simulink model "l1"  (R2016a)
settings: Solver=ode23  StartTime=0.0  StopTime=1000  RelTol=1e-10
settings Model: Creator=wojta  LastModifiedBy=wojta

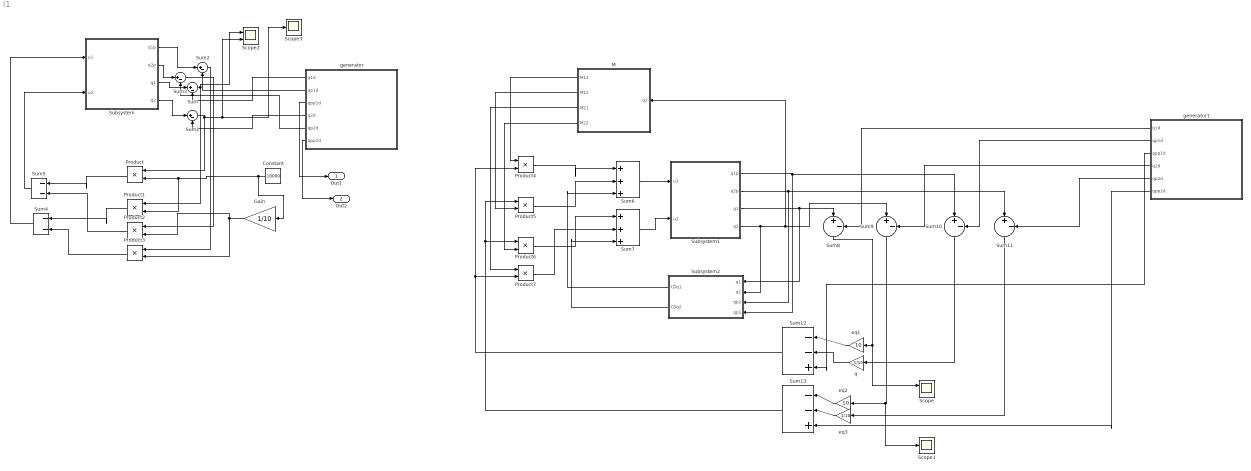
== system l1 ==
  Constant : Constant  Value=10000
  Gain : Gain  Gain=1/10
  M : Subsystem
  Product{,1..7} (8 alike) : Product
  Scope : Scope  NumInputPorts=2
  Scope1 : Scope
  Scope2 : Scope  NumInputPorts=2
  Scope3 : Scope
  Subsystem : Subsystem
  Subsystem1 : Subsystem
  Subsystem2 : Subsystem
  Sum{,1..3,8..11} (8 alike) : Sum  Inputs=|+-
  Sum12 : Sum  Inputs=|--+
  Sum13 : Sum  Inputs=|--+
  Sum4 : Sum  Inputs=|--
  Sum5 : Sum  Inputs=|--
  Sum6 : Sum  Inputs=|+++
  Sum7 : Sum  Inputs=|+++
  eq1 : Gain  Gain=10
  eq2 : Gain  Gain=10
  eq3 : Gain  Gain=1/10
  generator : Subsystem
  generator1 : Subsystem
  q : Gain  Gain=1/10
  Out1 : Outport
  Out2 : Outport  Port=2
  wires:
  Subsystem/3(q1) -> Sum/1
  generator/1(q1d) -> Sum/2
  Subsystem/4(q2) -> Sum1/1
  generator/4(q2d) -> Sum1/2
  Subsystem/1(q1p) -> Sum2/1
  generator/2(qp1d) -> Sum2/2
  Subsystem/2(q2p) -> Sum3/1
  generator/5(qp2d) -> Sum3/2
  Sum1/1 -> Scope2/2, Scope3/1, Product/1
  Sum/1 -> Product1/1, Scope2/1
  Constant/1 -> Gain/1, Product1/2, Product/2
  Sum3/1 -> Product2/1
  Sum2/1 -> Product3/1
  Gain/1 -> Product2/2, Product3/2
  Product2/1 -> Sum5/2
  Product/1 -> Sum5/1
  Product1/1 -> Sum4/1
  Product3/1 -> Sum4/2
  Sum5/1 -> Subsystem/2(u2)
  Sum4/1 -> Subsystem/1(u1)
  generator/3(qpp1d) -> Out1/1
  generator/6(qpp2d) -> Out2/1
  generator1/3(qpp1d) -> Sum12/3
  generator1/6(qpp2d) -> Sum13/3
  Subsystem1/4(q2) -> Subsystem2/2(q2), Sum9/1, M/1(q2)
  Sum12/1 -> Product4/2, Product7/2
  M/1(M11) -> Product4/1
  Sum13/1 -> Product5/1, Product6/1
  M/2(M12) -> Product5/2
  M/4(M22) -> Product6/2
  M/3(M21) -> Product7/1
  Sum6/1 -> Subsystem1/1(u1)
  Sum7/1 -> Subsystem1/2(u2)
  Product4/1 -> Sum6/1
  Product5/1 -> Sum6/2
  Product6/1 -> Sum7/1
  Product7/1 -> Sum7/2
  Subsystem2/1(CDq1) -> Sum6/3
  Subsystem2/2(CDq2) -> Sum7/3
  Subsystem1/1(q1p) -> Sum10/1, Subsystem2/4(qp1)
  Subsystem1/2(q2p) -> Sum11/1, Subsystem2/3(qp2)
  Subsystem1/3(q1) -> Sum8/1, Subsystem2/1(q1)
  generator1/1(q1d) -> Sum8/2
  generator1/4(q2d) -> Sum9/2
  generator1/2(qp1d) -> Sum10/2
  generator1/5(qp2d) -> Sum11/2
  eq1/1 -> Sum12/1
  q/1 -> Sum12/2
  Sum8/1 -> Scope/1, eq1/1
  Sum10/1 -> q/1
  eq2/1 -> Sum13/1
  eq3/1 -> Sum13/2
  Sum9/1 -> Scope1/1, eq2/1
  Sum11/1 -> eq3/1

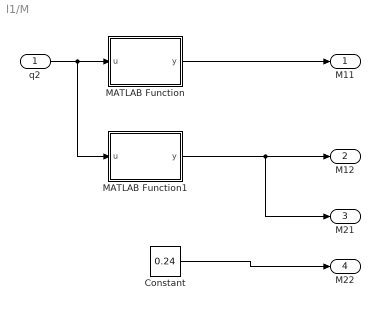
== system l1/M ==
  q2 : Inport
  Constant : Constant  Value=0.24
  MATLAB Function : MATLAB Function  TreatAsAtomicUnit=on
  MATLAB Function1 : MATLAB Function  TreatAsAtomicUnit=on
  M11 : Outport
  M12 : Outport  Port=2
  M21 : Outport  Port=3
  M22 : Outport  Port=4
  wires:
  q2/1 -> MATLAB Function1/1(u), MATLAB Function/1(u)
  MATLAB Function/1(y) -> M11/1
  MATLAB Function1/1(y) -> M21/1, M12/1
  Constant/1 -> M22/1

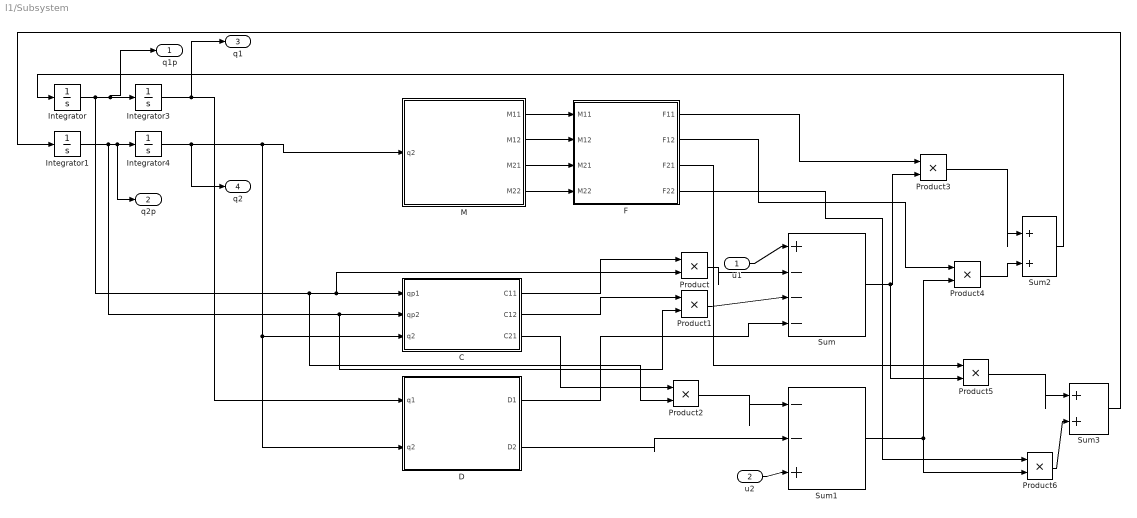
== system l1/Subsystem ==
  u1 : Inport
  u2 : Inport  Port=2
  C : Subsystem
  D : Subsystem
  F : Subsystem
  Integrator{,1,3..4} (4 alike) : Integrator
  M : Subsystem
  Product{,1..6} (7 alike) : Product
  Sum : Sum  Inputs=|+---
  Sum1 : Sum  Inputs=|--+
  Sum2 : Sum  Inputs=|++
  Sum3 : Sum  Inputs=|++
  q1p : Outport
  q2p : Outport  Port=2
  q1 : Outport  Port=3
  q2 : Outport  Port=4
  wires:
  Product6/1 -> Sum3/2
  F/3(F21) -> Product5/1
  Sum3/1 -> Integrator1/1
  Integrator/1 -> Product2/2, Product/2, C/1(qp1), q1p/1, Integrator3/1
  Integrator1/1 -> Product1/2, C/2(qp2), q2p/1, Integrator4/1
  Sum2/1 -> Integrator/1
  Integrator4/1 -> q2/1, D/2(q2), C/3(q2), M/1(q2)
  D/2(D2) -> Sum1/2
  Product4/1 -> Sum2/2
  C/1(C11) -> Product/1
  D/1(D1) -> Sum/4
  C/3(C21) -> Product2/1
  C/2(C12) -> Product1/1
  Sum/1 -> Product5/2, Product3/2
  F/2(F12) -> Product4/1
  F/1(F11) -> Product3/1
  M/2(M12) -> F/2(M12)
  M/1(M11) -> F/1(M11)
  M/4(M22) -> F/4(M22)
  Product2/1 -> Sum1/1
  Product1/1 -> Sum/3
  M/3(M21) -> F/3(M21)
  u2/1 -> Sum1/3
  Product/1 -> Sum/2
  Integrator3/1 -> q1/1, D/1(q1)
  u1/1 -> Sum/1
  Sum1/1 -> Product4/2, Product6/2
  Product5/1 -> Sum3/1
  F/4(F22) -> Product6/1
  Product3/1 -> Sum2/1

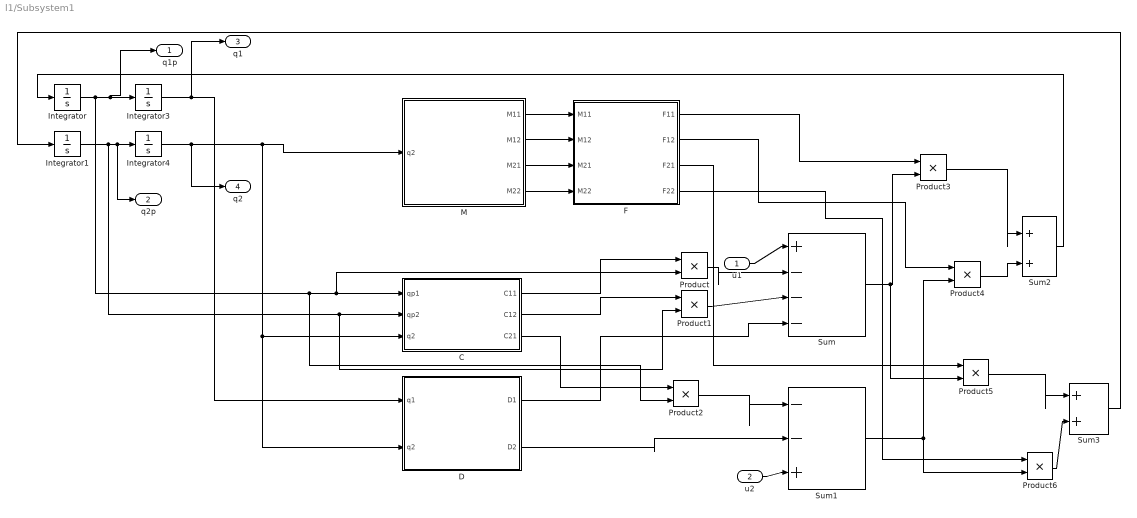
== system l1/Subsystem1 ==
  u1 : Inport
  u2 : Inport  Port=2
  C : Subsystem
  D : Subsystem
  F : Subsystem
  Integrator{,1,3..4} (4 alike) : Integrator
  M : Subsystem
  Product{,1..6} (7 alike) : Product
  Sum : Sum  Inputs=|+---
  Sum1 : Sum  Inputs=|--+
  Sum2 : Sum  Inputs=|++
  Sum3 : Sum  Inputs=|++
  q1p : Outport
  q2p : Outport  Port=2
  q1 : Outport  Port=3
  q2 : Outport  Port=4
  wires:
  Product6/1 -> Sum3/2
  F/3(F21) -> Product5/1
  Sum3/1 -> Integrator1/1
  Integrator/1 -> Product2/2, Product/2, C/1(qp1), q1p/1, Integrator3/1
  Integrator1/1 -> Product1/2, C/2(qp2), q2p/1, Integrator4/1
  Sum2/1 -> Integrator/1
  Integrator4/1 -> q2/1, D/2(q2), C/3(q2), M/1(q2)
  D/2(D2) -> Sum1/2
  Product4/1 -> Sum2/2
  C/1(C11) -> Product/1
  D/1(D1) -> Sum/4
  C/3(C21) -> Product2/1
  C/2(C12) -> Product1/1
  Sum/1 -> Product5/2, Product3/2
  F/2(F12) -> Product4/1
  F/1(F11) -> Product3/1
  M/2(M12) -> F/2(M12)
  M/1(M11) -> F/1(M11)
  M/4(M22) -> F/4(M22)
  Product2/1 -> Sum1/1
  Product1/1 -> Sum/3
  M/3(M21) -> F/3(M21)
  u2/1 -> Sum1/3
  Product/1 -> Sum/2
  Integrator3/1 -> q1/1, D/1(q1)
  u1/1 -> Sum/1
  Sum1/1 -> Product4/2, Product6/2
  Product5/1 -> Sum3/1
  F/4(F22) -> Product6/1
  Product3/1 -> Sum2/1

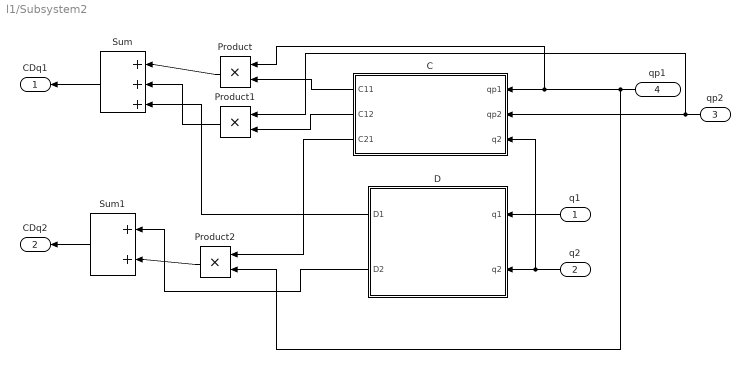
== system l1/Subsystem2 ==
  q1 : Inport
  q2 : Inport  Port=2
  qp2 : Inport  Port=3
  qp1 : Inport  Port=4
  C : Subsystem
  D : Subsystem
  Product : Product
  Product1 : Product
  Product2 : Product
  Sum : Sum  Inputs=|+++
  Sum1 : Sum  Inputs=|++
  CDq1 : Outport
  CDq2 : Outport  Port=2
  wires:
  q1/1 -> D/1(q1)
  q2/1 -> C/3(q2), D/2(q2)
  qp2/1 -> Product1/1, C/2(qp2)
  qp1/1 -> Product/1, C/1(qp1), Product2/2
  Sum1/1 -> CDq2/1
  Sum/1 -> CDq1/1
  Product/1 -> Sum/1
  Product1/1 -> Sum/2
  Product2/1 -> Sum1/2
  D/2(D2) -> Sum1/1
  D/1(D1) -> Sum/3
  C/1(C11) -> Product/2
  C/2(C12) -> Product1/2
  C/3(C21) -> Product2/1

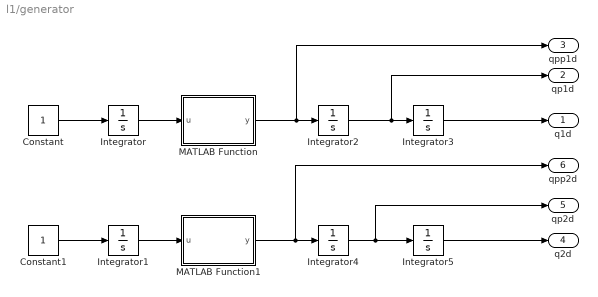
== system l1/generator ==
  Constant : Constant
  Constant1 : Constant
  Integrator{,1,3..4} (4 alike) : Integrator
  Integrator2 : Integrator  InitialCondition=0.5
  Integrator5 : Integrator  InitialCondition=2
  MATLAB Function : MATLAB Function  TreatAsAtomicUnit=on
  MATLAB Function1 : MATLAB Function  TreatAsAtomicUnit=on
  q1d : Outport
  qp1d : Outport  Port=2
  qpp1d : Outport  Port=3
  q2d : Outport  Port=4
  qp2d : Outport  Port=5
  qpp2d : Outport  Port=6
  wires:
  Constant/1 -> Integrator/1
  Integrator/1 -> MATLAB Function/1(u)
  Constant1/1 -> Integrator1/1
  Integrator1/1 -> MATLAB Function1/1(u)
  MATLAB Function/1(y) -> qpp1d/1, Integrator2/1
  Integrator2/1 -> qp1d/1, Integrator3/1
  Integrator4/1 -> qp2d/1, Integrator5/1
  Integrator3/1 -> q1d/1
  Integrator5/1 -> q2d/1
  MATLAB Function1/1(y) -> qpp2d/1, Integrator4/1

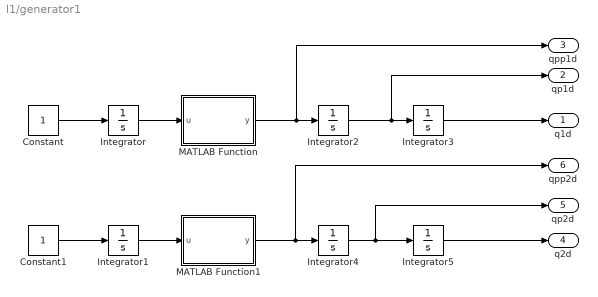
== system l1/generator1 ==
  Constant : Constant
  Constant1 : Constant
  Integrator{,1,3..4} (4 alike) : Integrator
  Integrator2 : Integrator  InitialCondition=0.5
  Integrator5 : Integrator  InitialCondition=2
  MATLAB Function : MATLAB Function  TreatAsAtomicUnit=on
  MATLAB Function1 : MATLAB Function  TreatAsAtomicUnit=on
  q1d : Outport
  qp1d : Outport  Port=2
  qpp1d : Outport  Port=3
  q2d : Outport  Port=4
  qp2d : Outport  Port=5
  qpp2d : Outport  Port=6
  wires:
  Constant/1 -> Integrator/1
  Integrator/1 -> MATLAB Function/1(u)
  Constant1/1 -> Integrator1/1
  Integrator1/1 -> MATLAB Function1/1(u)
  MATLAB Function/1(y) -> qpp1d/1, Integrator2/1
  Integrator2/1 -> qp1d/1, Integrator3/1
  Integrator4/1 -> qp2d/1, Integrator5/1
  Integrator3/1 -> q1d/1
  Integrator5/1 -> q2d/1
  MATLAB Function1/1(y) -> qpp2d/1, Integrator4/1

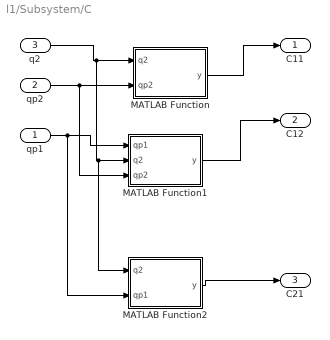
== system l1/Subsystem/C ==
  qp1 : Inport
  qp2 : Inport  Port=2
  q2 : Inport  Port=3
  MATLAB Function : MATLAB Function  TreatAsAtomicUnit=on
  MATLAB Function1 : MATLAB Function  TreatAsAtomicUnit=on
  MATLAB Function2 : MATLAB Function  TreatAsAtomicUnit=on
  C11 : Outport
  C12 : Outport  Port=2
  C21 : Outport  Port=3
  wires:
  MATLAB Function/1(y) -> C11/1
  qp2/1 -> MATLAB Function1/3(qp2), MATLAB Function/2(qp2)
  q2/1 -> MATLAB Function2/1(q2), MATLAB Function1/2(q2), MATLAB Function/1(q2)
  MATLAB Function1/1(y) -> C12/1
  qp1/1 -> MATLAB Function2/2(qp1), MATLAB Function1/1(qp1)
  MATLAB Function2/1(y) -> C21/1

== system l1/Subsystem/D ==
  q1 : Inport
  q2 : Inport  Port=2
  MATLAB Function : MATLAB Function  TreatAsAtomicUnit=on
  MATLAB Function1 : MATLAB Function  TreatAsAtomicUnit=on
  D1 : Outport
  D2 : Outport  Port=2
  wires:
  MATLAB Function/1(y) -> D1/1
  MATLAB Function1/1(y) -> D2/1
  q1/1 -> MATLAB Function1/1(q1), MATLAB Function/1(q1)
  q2/1 -> MATLAB Function1/2(q2), MATLAB Function/2(q2)

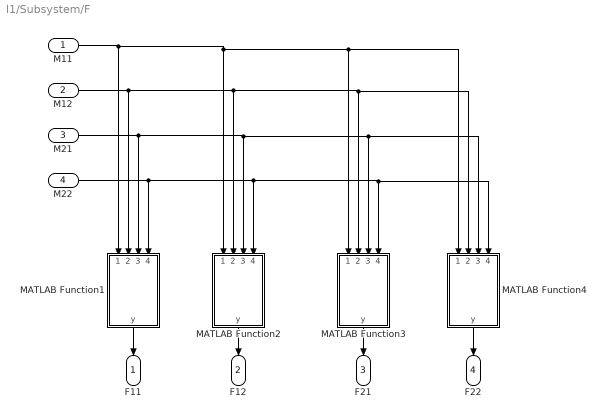
== system l1/Subsystem/F ==
  M11 : Inport
  M12 : Inport  Port=2
  M21 : Inport  Port=3
  M22 : Inport  Port=4
  MATLAB Function1 : MATLAB Function  TreatAsAtomicUnit=on
  MATLAB Function2 : MATLAB Function  TreatAsAtomicUnit=on
  MATLAB Function3 : MATLAB Function  TreatAsAtomicUnit=on
  MATLAB Function4 : MATLAB Function  TreatAsAtomicUnit=on
  F11 : Outport
  F12 : Outport  Port=2
  F21 : Outport  Port=3
  F22 : Outport  Port=4
  wires:
  MATLAB Function1/1(y) -> F11/1
  MATLAB Function2/1(y) -> F12/1
  MATLAB Function3/1(y) -> F21/1
  M11/1 -> MATLAB Function4/1(m11), MATLAB Function3/1(m11), MATLAB Function2/1(m11), MATLAB Function1/1(m11)
  M12/1 -> MATLAB Function4/2(m12), MATLAB Function3/2(m12), MATLAB Function2/2(m12), MATLAB Function1/2(m12)
  M21/1 -> MATLAB Function4/3(m21), MATLAB Function3/3(m21), MATLAB Function2/3(m21), MATLAB Function1/3(m21)
  M22/1 -> MATLAB Function4/4(m22), MATLAB Function3/4(m22), MATLAB Function2/4(m22), MATLAB Function1/4(m22)
  MATLAB Function4/1(y) -> F22/1

== system l1/Subsystem/M ==
  q2 : Inport
  Constant : Constant  Value=0.24
  MATLAB Function : MATLAB Function  TreatAsAtomicUnit=on
  MATLAB Function1 : MATLAB Function  TreatAsAtomicUnit=on
  M11 : Outport
  M12 : Outport  Port=2
  M21 : Outport  Port=3
  M22 : Outport  Port=4
  wires:
  q2/1 -> MATLAB Function1/1(u), MATLAB Function/1(u)
  MATLAB Function/1(y) -> M11/1
  MATLAB Function1/1(y) -> M21/1, M12/1
  Constant/1 -> M22/1

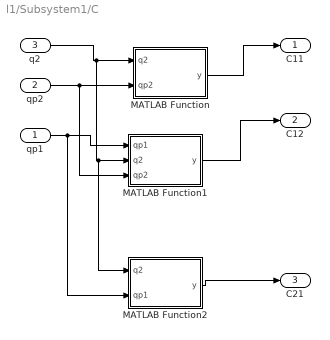
== system l1/Subsystem1/C ==
  qp1 : Inport
  qp2 : Inport  Port=2
  q2 : Inport  Port=3
  MATLAB Function : MATLAB Function  TreatAsAtomicUnit=on
  MATLAB Function1 : MATLAB Function  TreatAsAtomicUnit=on
  MATLAB Function2 : MATLAB Function  TreatAsAtomicUnit=on
  C11 : Outport
  C12 : Outport  Port=2
  C21 : Outport  Port=3
  wires:
  MATLAB Function/1(y) -> C11/1
  qp2/1 -> MATLAB Function1/3(qp2), MATLAB Function/2(qp2)
  q2/1 -> MATLAB Function2/1(q2), MATLAB Function1/2(q2), MATLAB Function/1(q2)
  MATLAB Function1/1(y) -> C12/1
  qp1/1 -> MATLAB Function2/2(qp1), MATLAB Function1/1(qp1)
  MATLAB Function2/1(y) -> C21/1

== system l1/Subsystem1/D ==
  q1 : Inport
  q2 : Inport  Port=2
  MATLAB Function : MATLAB Function  TreatAsAtomicUnit=on
  MATLAB Function1 : MATLAB Function  TreatAsAtomicUnit=on
  D1 : Outport
  D2 : Outport  Port=2
  wires:
  MATLAB Function/1(y) -> D1/1
  MATLAB Function1/1(y) -> D2/1
  q1/1 -> MATLAB Function1/1(q1), MATLAB Function/1(q1)
  q2/1 -> MATLAB Function1/2(q2), MATLAB Function/2(q2)

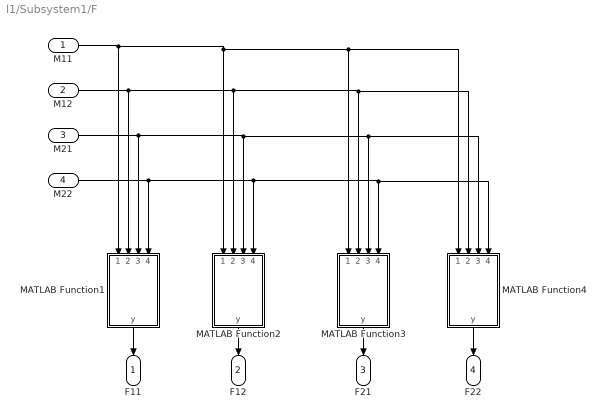
== system l1/Subsystem1/F ==
  M11 : Inport
  M12 : Inport  Port=2
  M21 : Inport  Port=3
  M22 : Inport  Port=4
  MATLAB Function1 : MATLAB Function  TreatAsAtomicUnit=on
  MATLAB Function2 : MATLAB Function  TreatAsAtomicUnit=on
  MATLAB Function3 : MATLAB Function  TreatAsAtomicUnit=on
  MATLAB Function4 : MATLAB Function  TreatAsAtomicUnit=on
  F11 : Outport
  F12 : Outport  Port=2
  F21 : Outport  Port=3
  F22 : Outport  Port=4
  wires:
  MATLAB Function1/1(y) -> F11/1
  MATLAB Function2/1(y) -> F12/1
  MATLAB Function3/1(y) -> F21/1
  M11/1 -> MATLAB Function4/1(m11), MATLAB Function3/1(m11), MATLAB Function2/1(m11), MATLAB Function1/1(m11)
  M12/1 -> MATLAB Function4/2(m12), MATLAB Function3/2(m12), MATLAB Function2/2(m12), MATLAB Function1/2(m12)
  M21/1 -> MATLAB Function4/3(m21), MATLAB Function3/3(m21), MATLAB Function2/3(m21), MATLAB Function1/3(m21)
  M22/1 -> MATLAB Function4/4(m22), MATLAB Function3/4(m22), MATLAB Function2/4(m22), MATLAB Function1/4(m22)
  MATLAB Function4/1(y) -> F22/1

== system l1/Subsystem1/M ==
  q2 : Inport
  Constant : Constant  Value=0.24
  MATLAB Function : MATLAB Function  TreatAsAtomicUnit=on
  MATLAB Function1 : MATLAB Function  TreatAsAtomicUnit=on
  M11 : Outport
  M12 : Outport  Port=2
  M21 : Outport  Port=3
  M22 : Outport  Port=4
  wires:
  q2/1 -> MATLAB Function1/1(u), MATLAB Function/1(u)
  MATLAB Function/1(y) -> M11/1
  MATLAB Function1/1(y) -> M21/1, M12/1
  Constant/1 -> M22/1

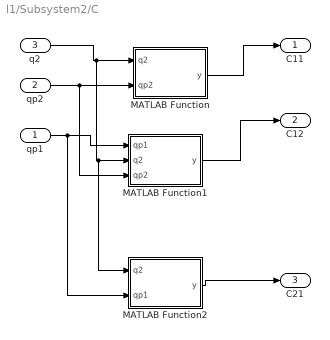
== system l1/Subsystem2/C ==
  qp1 : Inport
  qp2 : Inport  Port=2
  q2 : Inport  Port=3
  MATLAB Function : MATLAB Function  TreatAsAtomicUnit=on
  MATLAB Function1 : MATLAB Function  TreatAsAtomicUnit=on
  MATLAB Function2 : MATLAB Function  TreatAsAtomicUnit=on
  C11 : Outport
  C12 : Outport  Port=2
  C21 : Outport  Port=3
  wires:
  MATLAB Function/1(y) -> C11/1
  qp2/1 -> MATLAB Function1/3(qp2), MATLAB Function/2(qp2)
  q2/1 -> MATLAB Function2/1(q2), MATLAB Function1/2(q2), MATLAB Function/1(q2)
  MATLAB Function1/1(y) -> C12/1
  qp1/1 -> MATLAB Function2/2(qp1), MATLAB Function1/1(qp1)
  MATLAB Function2/1(y) -> C21/1

== system l1/Subsystem2/D ==
  q1 : Inport
  q2 : Inport  Port=2
  MATLAB Function : MATLAB Function  TreatAsAtomicUnit=on
  MATLAB Function1 : MATLAB Function  TreatAsAtomicUnit=on
  D1 : Outport
  D2 : Outport  Port=2
  wires:
  MATLAB Function/1(y) -> D1/1
  MATLAB Function1/1(y) -> D2/1
  q1/1 -> MATLAB Function1/1(q1), MATLAB Function/1(q1)
  q2/1 -> MATLAB Function1/2(q2), MATLAB Function/2(q2)

== matlab function l1/Subsystem/M/MATLAB Function1 ==
  data: u input; y output
function y = fcn(u)
%#codegen

y = 0.24+0.231*cos(u);

== matlab function l1/Subsystem/M/MATLAB Function ==
  data: u input; y output
function y = fcn(u)
%#codegen

y = 3.1+0.462*cos(u);

== matlab function l1/Subsystem/C/MATLAB Function ==
  data: q2 input; y output; qp2 input
function y = fcn(q2, qp2)
%#codegen

y = -0.231*sin(q2)*qp2;

== matlab function l1/Subsystem/C/MATLAB Function1 ==
  data: qp1 input; y output; q2 input; qp2 input
function y = fcn(qp1, q2, qp2)
%#codegen

y = -0.231*sin(q2)*(qp1+qp2);

== matlab function l1/Subsystem/C/MATLAB Function2 ==
  data: q2 input; y output; qp1 input
function y = fcn(q2, qp1)
%#codegen

y = 0.231*sin(q2)*qp1;

== matlab function l1/Subsystem/D/MATLAB Function ==
  data: q1 input; y output; q2 input
function y = fcn(q1, q2)
%#codegen

y = 9.81*(9.5*cos(q1)+0.77*cos(q1+q2));

== matlab function l1/Subsystem/D/MATLAB Function1 ==
  data: q1 input; y output; q2 input
function y = fcn(q1, q2)
%#codegen

y = 9.81*0.77*cos(q1+q2);

== matlab function l1/generator/MATLAB Function ==
  data: u input; y output
function y = fcn(u)
%#codegen

y = -0.5*sin(u);

== matlab function l1/Subsystem/F/MATLAB Function1 ==
  data: m11 input; y output; m12 input; m21 input; m22 input
function y = fcn(m11, m12, m21, m22)
%#codegen

y = m22/(m11*m22-m12*m21);

== matlab function l1/Subsystem/F/MATLAB Function2 ==
  data: m11 input; y output; m12 input; m21 input; m22 input
function y = fcn(m11, m12, m21, m22)
%#codegen

y = -m12/(m11*m22-m12*m21);

== matlab function l1/Subsystem/F/MATLAB Function3 ==
  data: m11 input; y output; m12 input; m21 input; m22 input
function y = fcn(m11, m12, m21, m22)
%#codegen

y = -m21/(m11*m22-m12*m21);

== matlab function l1/Subsystem/F/MATLAB Function4 ==
  data: m11 input; y output; m12 input; m21 input; m22 input
function y = fcn(m11, m12, m21, m22)
%#codegen

y = m11/(m11*m22-m12*m21);

== matlab function l1/generator/MATLAB Function1 ==
  data: u input; y output
function y = fcn(u)
%#codegen

y = -8*cos(2*u);

== matlab function l1/Subsystem1/C/MATLAB Function ==
  data: q2 input; y output; qp2 input
function y = fcn(q2, qp2)
%#codegen

y = -0.231*sin(q2)*qp2;

== matlab function l1/Subsystem1/C/MATLAB Function1 ==
  data: qp1 input; y output; q2 input; qp2 input
function y = fcn(qp1, q2, qp2)
%#codegen

y = -0.231*sin(q2)*(qp1+qp2);

== matlab function l1/Subsystem1/C/MATLAB Function2 ==
  data: q2 input; y output; qp1 input
function y = fcn(q2, qp1)
%#codegen

y = 0.231*sin(q2)*qp1;

== matlab function l1/Subsystem1/D/MATLAB Function ==
  data: q1 input; y output; q2 input
function y = fcn(q1, q2)
%#codegen

y = 9.81*(9.5*cos(q1)+0.77*cos(q1+q2));

== matlab function l1/Subsystem1/D/MATLAB Function1 ==
  data: q1 input; y output; q2 input
function y = fcn(q1, q2)
%#codegen

y = 9.81*0.77*cos(q1+q2);

== matlab function l1/Subsystem1/F/MATLAB Function1 ==
  data: m11 input; y output; m12 input; m21 input; m22 input
function y = fcn(m11, m12, m21, m22)
%#codegen

y = m22/(m11*m22-m12*m21);

== matlab function l1/Subsystem1/F/MATLAB Function2 ==
  data: m11 input; y output; m12 input; m21 input; m22 input
function y = fcn(m11, m12, m21, m22)
%#codegen

y = -m12/(m11*m22-m12*m21);

== matlab function l1/Subsystem1/F/MATLAB Function3 ==
  data: m11 input; y output; m12 input; m21 input; m22 input
function y = fcn(m11, m12, m21, m22)
%#codegen

y = -m21/(m11*m22-m12*m21);

== matlab function l1/Subsystem1/F/MATLAB Function4 ==
  data: m11 input; y output; m12 input; m21 input; m22 input
function y = fcn(m11, m12, m21, m22)
%#codegen

y = m11/(m11*m22-m12*m21);

== matlab function l1/Subsystem1/M/MATLAB Function ==
  data: u input; y output
function y = fcn(u)
%#codegen

y = 3.1+0.462*cos(u);

== matlab function l1/Subsystem1/M/MATLAB Function1 ==
  data: u input; y output
function y = fcn(u)
%#codegen

y = 0.24+0.231*cos(u);

== matlab function l1/generator1/MATLAB Function ==
  data: u input; y output
function y = fcn(u)
%#codegen

y = -0.5*sin(u);

== matlab function l1/generator1/MATLAB Function1 ==
  data: u input; y output
function y = fcn(u)
%#codegen

y = -8*cos(2*u);

== matlab function l1/M/MATLAB Function ==
  data: u input; y output
function y = fcn(u)
%#codegen

y = 3.1+0.462*cos(u);

== matlab function l1/M/MATLAB Function1 ==
  data: u input; y output
function y = fcn(u)
%#codegen

y = 0.24+0.231*cos(u);

== matlab function l1/Subsystem2/C/MATLAB Function ==
  data: q2 input; y output; qp2 input
function y = fcn(q2, qp2)
%#codegen

y = -0.231*sin(q2)*qp2;

== matlab function l1/Subsystem2/C/MATLAB Function1 ==
  data: qp1 input; y output; q2 input; qp2 input
function y = fcn(qp1, q2, qp2)
%#codegen

y = -0.231*sin(q2)*(qp1+qp2);

== matlab function l1/Subsystem2/C/MATLAB Function2 ==
  data: q2 input; y output; qp1 input
function y = fcn(q2, qp1)
%#codegen

y = 0.231*sin(q2)*qp1;

== matlab function l1/Subsystem2/D/MATLAB Function ==
  data: q1 input; y output; q2 input
function y = fcn(q1, q2)
%#codegen

y = 9.81*(9.5*cos(q1)+0.77*cos(q1+q2));

== matlab function l1/Subsystem2/D/MATLAB Function1 ==
  data: q1 input; y output; q2 input
function y = fcn(q1, q2)
%#codegen

y = 9.81*0.77*cos(q1+q2);
